simulink model "CRDI_Integrated_Model0707"  (R2019a)
settings: configuration reference "cs1" (kept outside this file)
PreLoadFcn:
  | Configaration_Setting
undefined symbols (not defined in the file or in its folder): AreaOfOrifice_Constant, CcConstant_0, CcConstant_1, Constant_0, Constant_1, Constant_One, Divide_by_100, Error_code_101, Error_code_102, FilterConstant_0, FilterConstant_1, FilterConstant_100, FilterConstant_5, FilterConstant_50, Final_Crank_Angle, Fuel_Discharge, HPPConstant1, HPPConstant2, LPPConstant_0, LPPConstant_1, LPPConstant_10, LPPConstant_3, Main_TgrAng_Inj1, Main_TgrAng_Inj2, Main_TgrAng_Inj3, Main_TgrAng_Inj4, MeterToLiter_Conversion, Orifice_Diameter, Percentage, Pi_value, Post_TgrAng_Inj1, Post_TgrAng_Inj2, Post_TgrAng_Inj3, Post_TgrAng_Inj4, Pre_TgrAng_Inj1, Pre_TgrAng_Inj2, Pre_TgrAng_Inj3, Pre_TgrAng_Inj4, Re_Rounding_Constant, Required_PulseConstant1, Required_PulseConstant2, Required_PulseConstant3, Required_PulseConstant4, resistance_constant, Rounding_Constant_100, Scalling_Factor, Unit_Angle_Compare, Velocity_MulFactor1, Velocity_MulFactor2, Velocity_MulFactor3, Zero_Pulse
libraries: simulink x4
(part 1 of 2)
settings Model: DataDictionary=CRDI_Integrated_Model.sldd  EnableAccessToBaseWorkspace=off  Creator=ADVAIT ELECTRICALS  LastModifiedBy=user
settings ConfigSetRef: SourceName=cs1

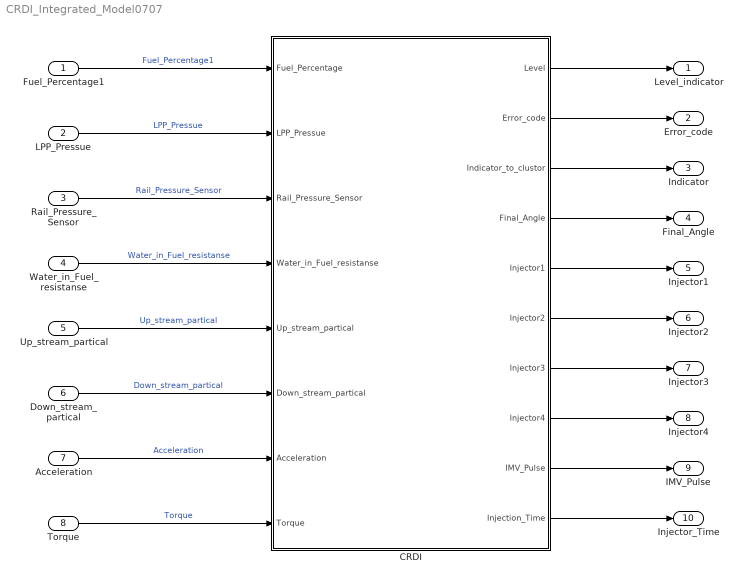
== system CRDI_Integrated_Model0707 ==
  Fuel_Percentage1 : Inport
  LPP_Pressue : Inport  Port=2
  Rail_Pressure_Sensor : Inport  Port=3
  Water_in_Fuel_resistanse : Inport  Port=4
  Up_stream_partical : Inport  Port=5
  Down_stream_partical : Inport  Port=6
  Acceleration : Inport  Port=7
  Torque : Inport  Port=8
  CRDI : Subsystem  TreatAsAtomicUnit=on
  Level_indicator : Outport
  Error_code : Outport  Port=2
  Indicator : Outport  Port=3
  Final_Angle : Outport  Port=4
  Injector1 : Outport  Port=5
  Injector2 : Outport  Port=6
  Injector3 : Outport  Port=7
  Injector4 : Outport  Port=8
  IMV_Pulse : Outport  Port=9
  Injector_Time : Outport  Port=10
  wires:
  LPP_Pressue/1 -> CRDI/2(LPP_Pressue)  "LPP_Pressue"
  Fuel_Percentage1/1 -> CRDI/1(Fuel_Percentage)  "Fuel_Percentage1"
  Rail_Pressure_Sensor/1 -> CRDI/3(Rail_Pressure_Sensor)  "Rail_Pressure_Sensor"
  Up_stream_partical/1 -> CRDI/5(Up_stream_partical)  "Up_stream_partical"
  Water_in_Fuel_resistanse/1 -> CRDI/4(Water_in_Fuel_resistanse)  "Water_in_Fuel_resistanse"
  Down_stream_partical/1 -> CRDI/6(Down_stream_partical)  "Down_stream_partical"
  CRDI/1(Level) -> Level_indicator/1
  CRDI/2(Error_code) -> Error_code/1
  CRDI/3(Indicator_to_clustor) -> Indicator/1
  CRDI/6(Injector2) -> Injector2/1
  CRDI/5(Injector1) -> Injector1/1
  CRDI/4(Final_Angle) -> Final_Angle/1
  CRDI/9(IMV_Pulse) -> IMV_Pulse/1
  CRDI/10(Injection_Time) -> Injector_Time/1
  CRDI/8(Injector4) -> Injector4/1
  CRDI/7(Injector3) -> Injector3/1
  Acceleration/1 -> CRDI/7(Acceleration)  "Acceleration"
  Torque/1 -> CRDI/8(Torque)  "Torque"

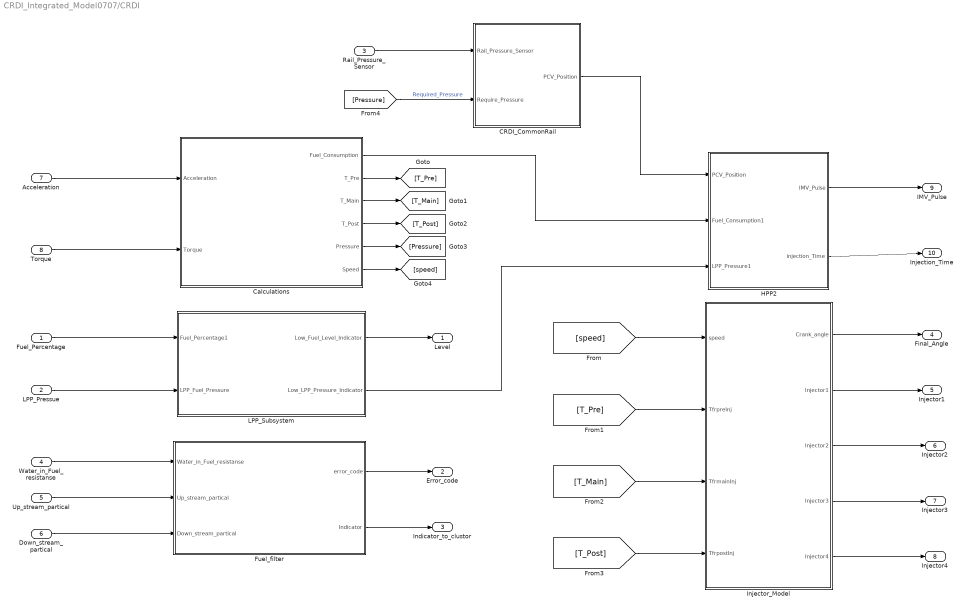
== system CRDI_Integrated_Model0707/CRDI ==
  Fuel_Percentage : Inport
  LPP_Pressue : Inport  Port=2
  Rail_Pressure_Sensor : Inport  Port=3
  Water_in_Fuel_resistanse : Inport  Port=4
  Up_stream_partical : Inport  Port=5
  Down_stream_partical : Inport  Port=6
  Acceleration : Inport  Port=7
  Torque : Inport  Port=8
  CRDI_CommonRail : Subsystem  TreatAsAtomicUnit=on
  Calculations : Subsystem
  Fuel_filter : Subsystem  TreatAsAtomicUnit=on
  HPP2 : Subsystem
  Injector_Model : Subsystem  TreatAsAtomicUnit=on
  LPP_Subsystem : Subsystem  TreatAsAtomicUnit=on
  Level : Outport
  Error_code : Outport  Port=2
  Indicator_to_clustor : Outport  Port=3
  Final_Angle : Outport  Port=4
  Injector1 : Outport  Port=5
  Injector2 : Outport  Port=6
  Injector3 : Outport  Port=7
  Injector4 : Outport  Port=8
  IMV_Pulse : Outport  Port=9
  Injection_Time : Outport  Port=10
  wires:
  CRDI_CommonRail/1(PCV_Position) -> HPP2/1(PCV_Position)
  Fuel_Percentage/1 -> LPP_Subsystem/1(Fuel_Percentage1)
  LPP_Subsystem/1(Low_Fuel_Level_Indicator) -> Level/1
  LPP_Pressue/1 -> LPP_Subsystem/2(LPP_Fuel_Pressure)
  Water_in_Fuel_resistanse/1 -> Fuel_filter/1(Water_in_Fuel_resistanse)
  Down_stream_partical/1 -> Fuel_filter/3(Down_stream_partical)
  Up_stream_partical/1 -> Fuel_filter/2(Up_stream_partical)
  Injector_Model/1(Crank_angle) -> Final_Angle/1
  Injector_Model/5(Injector4) -> Injector4/1
  Injector_Model/2(Injector1) -> Injector1/1
  Injector_Model/3(Injector2) -> Injector2/1
  Injector_Model/4(Injector3) -> Injector3/1
  [speed] -> Injector_Model/1(speed)
  Fuel_filter/1(error_code) -> Error_code/1
  Fuel_filter/2(Indicator) -> Indicator_to_clustor/1
  HPP2/2(injection_Time) -> Injection_Time/1
  HPP2/1(IMV_Pulse) -> IMV_Pulse/1
  LPP_Subsystem/2(Low_LPP_Pressure_Indicator) -> HPP2/3(LPP_Pressure1)
  [T_Pre] -> Injector_Model/2(TfrpreInj)
  [T_Main] -> Injector_Model/3(TfrmainInj)
  [T_Post] -> Injector_Model/4(TfrpostInj)
  Calculations/2(T_Pre) -> [T_Pre]
  Calculations/3(T_Main) -> [T_Main]
  Calculations/4(T_Post) -> [T_Post]
  Calculations/5(Pressure) -> [Pressure]
  Calculations/1(Fuel_Consumption) -> HPP2/2(Fuel_Consumption1)
  Calculations/6(Speed) -> [speed]
  [Pressure] -> CRDI_CommonRail/2(Require_Pressure)  "Required_Pressure"
  Rail_Pressure_Sensor/1 -> CRDI_CommonRail/1(Rail_Pressure_Sensor)
  Acceleration/1 -> Calculations/1(Acceleration)
  Torque/1 -> Calculations/2(Torque)

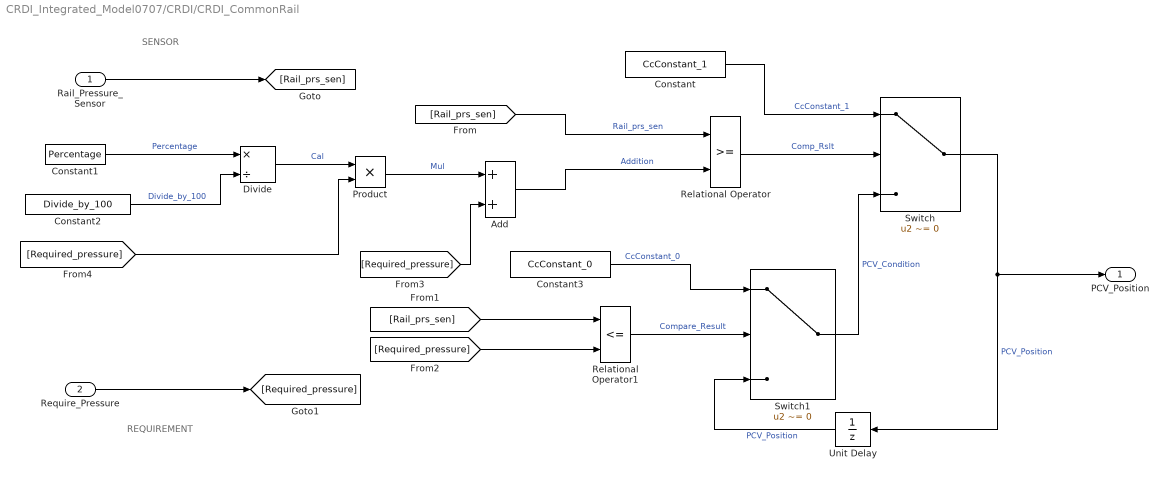
== system CRDI_Integrated_Model0707/CRDI/CRDI_CommonRail ==
  note: REQUIREMENT
  note: SENSOR
  Rail_Pressure_Sensor : Inport
  Require_Pressure : Inport  Port=2
  Add : Sum
  Constant : Constant  Value=CcConstant_1  OutDataTypeStr=boolean
  Constant1 : Constant  Value=Percentage
  Constant2 : Constant  Value=Divide_by_100
  Constant3 : Constant  Value=CcConstant_0  OutDataTypeStr=boolean
  Divide : Product  Inputs=*/  OutDataTypeStr=single
  Product : Product
  Relational Operator : RelationalOperator  OutDataTypeStr=boolean  RndMeth=Simplest
  Relational Operator1 : RelationalOperator  Operator=<=  OutDataTypeStr=boolean  RndMeth=Simplest
  Switch : Switch  Criteria=u2 ~= 0  OutDataTypeStr=boolean
  Switch1 : Switch  Criteria=u2 ~= 0  OutDataTypeStr=boolean
  Unit Delay : UnitDelay  SampleTime=-1  HasFrameUpgradeWarning=on
  PCV_Position : Outport
  wires:
  Constant/1 -> Switch/1  "CcConstant_1"
  Switch/1 -> PCV_Position/1, Unit Delay/1  "PCV_Position"
  Relational Operator/1 -> Switch/2  "Comp_Rslt"
  Unit Delay/1 -> Switch1/3  "PCV_Position"
  Switch1/1 -> Switch/3  "PCV_Condition"
  Product/1 -> Add/1  "Mul"
  Relational Operator1/1 -> Switch1/2  "Compare_Result"
  Add/1 -> Relational Operator/2  "Addition"
  Divide/1 -> Product/1  "Cal"
  Constant3/1 -> Switch1/1  "CcConstant_0"
  Constant1/1 -> Divide/1  "Percentage"
  Constant2/1 -> Divide/2  "Divide_by_100"
  [Rail_prs_sen] -> Relational Operator/1  "Rail_prs_sen"
  Rail_Pressure_Sensor/1 -> [Rail_prs_sen]
  [Rail_prs_sen] -> Relational Operator1/1
  Require_Pressure/1 -> [Required_pressure]
  [Required_pressure] -> Product/2
  [Required_pressure] -> Add/2
  [Required_pressure] -> Relational Operator1/2

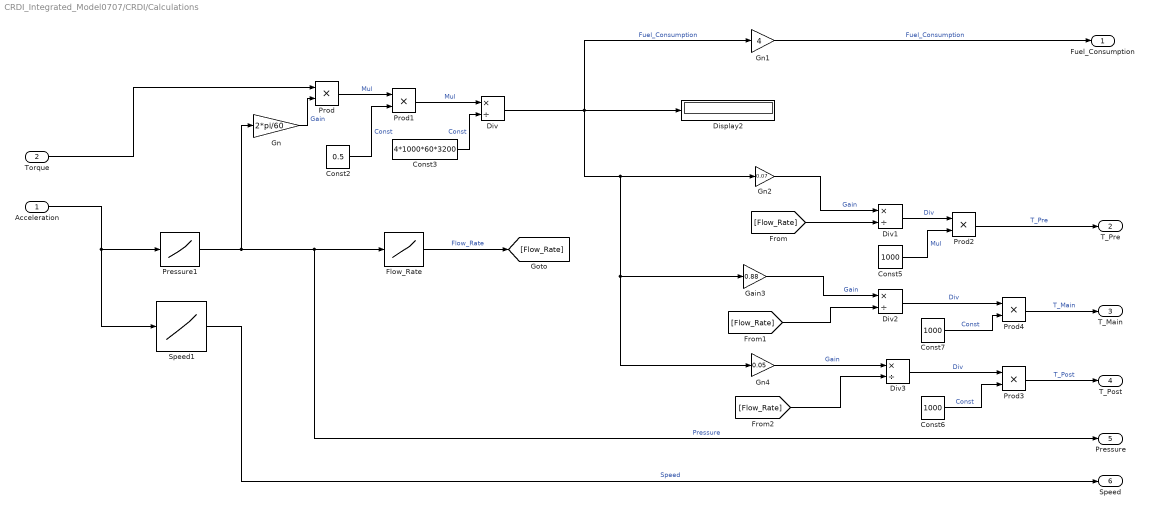
== system CRDI_Integrated_Model0707/CRDI/Calculations ==
  Acceleration : Inport
  Torque : Inport  Port=2
  Const2 : Constant  Value=0.5  OutDataTypeStr=single
  Const3 : Constant  Value=4*1000*60*3200  OutDataTypeStr=single
  Const5 : Constant  Value=1000
  Const6 : Constant  Value=1000  OutDataTypeStr=single
  Const7 : Constant  Value=1000  OutDataTypeStr=single
  Display2 : Display
  Div{,1..3} (4 alike) : Product  Inputs=*/  OutDataTypeStr=single
  Flow_Rate : Lookup_n-D  NumberOfTableDimensions=1  BreakpointsForDimension1=[300 450 600 750 900 1050 1200 1350 1500 1650 1800]  Table=|  InternalRulePriority=Speed  RndMeth=Simplest  InputSameDT=on
      | [0.04780543
      | 0.058549455
      | 0.067607087
      | 0.075587021
      | 0.082801433
      | 0.089435769
      | 0.095610859
      | 0.10141063
      | 0.10689619
      | 0.11211367
      | 0.11709891
      | ]
  Gain3 : Gain  Gain=0.88  OutDataTypeStr=single
  Gn : Gain  Gain=2*pi/60
  Gn1 : Gain  Gain=4  OutDataTypeStr=single
  Gn2 : Gain  Gain=0.07
  Gn4 : Gain  Gain=0.05  OutDataTypeStr=single
  Pressure1 : Lookup_n-D  NumberOfTableDimensions=1  BreakpointsForDimension1=[0 10 20 30 40 50 60 70 80 90 100]  Table=[300 450 600 750 900 1050 1200 1350 1500 1650 1800]  InternalRulePriority=Speed  RndMeth=Simplest  InputSameDT=on
  Prod{,1,3..4} (4 alike) : Product  OutDataTypeStr=single
  Prod2 : Product  OutDataTypeStr=single  SaturateOnIntegerOverflow=on
  Speed1 : Lookup_n-D  NumberOfTableDimensions=1  BreakpointsForDimension1=[0 10 20 30 40 50 60 70 80 90 100]  Table=[800 1040 1280 1520 1760 2000 2240 2480 2720 2960 3200]  InternalRulePriority=Speed  RndMeth=Simplest  InputSameDT=on
  Fuel_Consumption : Outport  OutDataTypeStr=single
  T_Pre : Outport  Port=2  OutDataTypeStr=single
  T_Main : Outport  Port=3  OutDataTypeStr=single
  T_Post : Outport  Port=4  OutDataTypeStr=single
  Pressure : Outport  Port=5  OutDataTypeStr=single
  Speed : Outport  Port=6
  wires:
  Prod/1 -> Prod1/1  "Mul"
  Div2/1 -> Prod4/1  "Div"
  Gn2/1 -> Div1/1  "Gain"
  Const6/1 -> Prod3/2  "Const"
  Pressure1/1 -> Pressure/1, Flow_Rate/1, Gn/1  "Pressure"
  Div/1 -> Gn1/1, Display2/1, Gn4/1, Gain3/1, Gn2/1  "Fuel_Consumption"
  Div3/1 -> Prod3/1  "Div"
  Const2/1 -> Prod1/2  "Const"
  Prod1/1 -> Div/1  "Mul"
  Gn4/1 -> Div3/1  "Gain"
  Const7/1 -> Prod4/2  "Const"
  Acceleration/1 -> Speed1/1, Pressure1/1
  Div1/1 -> Prod2/1  "Div"
  Gn1/1 -> Fuel_Consumption/1  "Fuel_Consumption"
  Prod3/1 -> T_Post/1  "T_Post"
  Prod2/1 -> T_Pre/1  "T_Pre"
  Const3/1 -> Div/2  "Const"
  Gn/1 -> Prod/2  "Gain"
  Const5/1 -> Prod2/2  "Mul"
  Prod4/1 -> T_Main/1  "T_Main"
  Gain3/1 -> Div2/1  "Gain"
  Torque/1 -> Prod/1
  Flow_Rate/1 -> [Flow_Rate]  "Flow_Rate"
  [Flow_Rate] -> Div1/2
  [Flow_Rate] -> Div2/2
  [Flow_Rate] -> Div3/2
  Speed1/1 -> Speed/1  "Speed"

== system CRDI_Integrated_Model0707/CRDI/Fuel_filter ==
  Water_in_Fuel_resistanse : Inport  OutDataTypeStr=single
  Up_stream_partical : Inport  Port=2  OutDataTypeStr=single
  Down_stream_partical : Inport  Port=3  OutDataTypeStr=single
  Calculation : Subsystem
  Condition : Subsystem
  Division_by_0 : Subsystem  TreatAsAtomicUnit=on
  Error_Signal : Subsystem  TreatAsAtomicUnit=on
  Error_code : Subsystem  TreatAsAtomicUnit=on
  On_Delay : Subsystem  TreatAsAtomicUnit=on
  On_delay : Subsystem  TreatAsAtomicUnit=on
  Switch_Condition : Subsystem
  division_by_0 : Subsystem  TreatAsAtomicUnit=on
  error_code : Outport  OutDataTypeStr=single
  Indicator : Outport  Port=2  OutDataTypeStr=boolean
  wires:
  Error_code/1(Error_code) -> error_code/1
  Error_Signal/1(indicator) -> Indicator/1  "Indicator"
  On_Delay/1(error) -> Error_Signal/1(water_error), Error_code/1(water_error)
  On_delay/1(Filter_error) -> Error_code/2(Filter_error), Error_Signal/2(filter_error)
  Down_stream_partical/1 -> Division_by_0/1(Down_stream_partical)
  Water_in_Fuel_resistanse/1 -> Switch_Condition/1(Fuel_Filter)
  Switch_Condition/1(Switch_condition) -> On_Delay/1(switch_condition)
  division_by_0/1(Switch_condition) -> Condition/2(Switch_Condition)
  Condition/1(condition) -> On_delay/1(Switch_condition)
  Up_stream_partical/1 -> Calculation/1(Up_stream_partical)
  Division_by_0/1(Downstream_partical) -> Calculation/2(Down_stream_partical)
  Calculation/1(Add) -> Condition/1(Ad)
  Calculation/2(product) -> division_by_0/1(Beeta_retio)

== system CRDI_Integrated_Model0707/CRDI/HPP2 ==
  PCV_Position : Inport  OutDataTypeStr=boolean
  Fuel_Consumption1 : Inport  Port=2  OutDataTypeStr=single  PortDimensions=1  SampleTime=[0.01,0]
  LPP_Pressure1 : Inport  Port=3  OutDataTypeStr=single  PortDimensions=1  SampleTime=[0.01,0]
  AreaOfOrifice : Subsystem  TreatAsAtomicUnit=on
  Injection_Time_Cal : Subsystem
  Input_Para : Subsystem
  PCV_Position_Action : Subsystem
  Required_Pulse : Subsystem  TreatAsAtomicUnit=on
  Rounding2 : Subsystem  TreatAsAtomicUnit=on
  Rounding3 : Subsystem  Commented=on  TreatAsAtomicUnit=on
  Subsystem1 : Subsystem  Commented=on
  Velocity : Subsystem  TreatAsAtomicUnit=on
  IMV_Pulse : Outport  OutDataTypeStr=boolean  PortDimensions=1  SampleTime=[0.01,0]
  injection_Time : Outport  Port=2  OutDataTypeStr=single  PortDimensions=1  SampleTime=[0.01,0]
  wires:
  Injection_Time_Cal/1(Injection_Time) -> Rounding2/1(In1)
  Fuel_Consumption1/1 -> Injection_Time_Cal/2(Fuel_Consumption)
  Velocity/1(Velocity) -> Input_Para/1(Velocity)
  LPP_Pressure1/1 -> Velocity/1(LPP_Pressurer1)
  Input_Para/1(Multiply11) -> Injection_Time_Cal/1(Flow_Rate)
  AreaOfOrifice/1(Orifice_Area) -> Input_Para/2(Orifice_Area)
  PCV_Position_Action/1(Injector_Time) -> injection_Time/1, Required_Pulse/1(On_Time)
  Rounding2/1(Rounding2) -> PCV_Position_Action/1(Injector_Time1)
  PCV_Position/1 -> PCV_Position_Action/2(PCV_Position)
  Required_Pulse/1(IMV_Pulse) -> IMV_Pulse/1

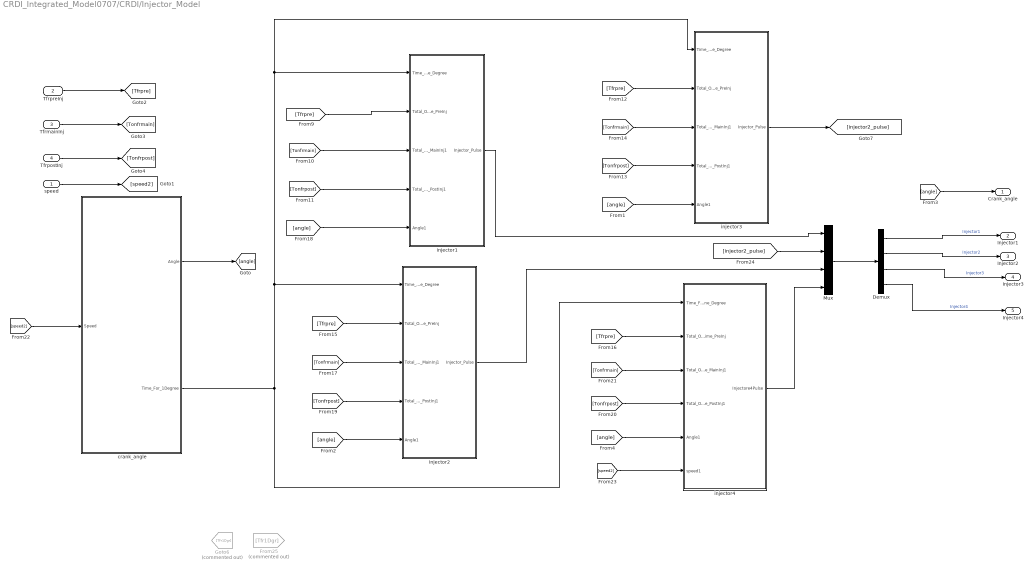
== system CRDI_Integrated_Model0707/CRDI/Injector_Model ==
  speed : Inport  OutDataTypeStr=single
  TfrpreInj : Inport  Port=2  OutDataTypeStr=single
  TfrmainInj : Inport  Port=3  OutDataTypeStr=single
  TfrpostInj : Inport  Port=4  OutDataTypeStr=single
  Demux : Demux
  From25 : From  Commented=on  GotoTag=Tfr1Dgr
  Goto6 : Goto  Commented=on  GotoTag=Tfr1Dgr
  Mux : Mux
  crank_angle : Subsystem  TreatAsAtomicUnit=on
  injector1 : Subsystem  TreatAsAtomicUnit=on
  injector2 : Subsystem  TreatAsAtomicUnit=on
  injector3 : Subsystem  TreatAsAtomicUnit=on
  injector4 : Subsystem  TreatAsAtomicUnit=on
  Crank_angle : Outport
  Injector1 : Outport  Port=2
  Injector2 : Outport  Port=3
  Injector3 : Outport  Port=4
  Injector4 : Outport  Port=5
  wires:
  [Tfrpre] -> injector3/2(Total_On_Time_PreInj)
  [angle] -> injector1/5(Angle1)
  [Tonfrmain] -> injector1/3(Total_On_Time_MainInj1)
  [angle] -> injector4/5(Angle1)
  TfrmainInj/1 -> [Tonfrmain]
  [Tonfrpost] -> injector3/4(Total_On_Time_PostInj1)
  [Tonfrmain] -> injector2/3(Total_On_Time_MainInj1)
  [Tonfrmain] -> injector4/3(Total_On_Time_MainInj1)
  TfrpostInj/1 -> [Tonfrpost]
  [Tfrpre] -> injector2/2(Total_On_Time_PreInj)
  crank_angle/1(Angle) -> [angle]
  crank_angle/2(Time_For_1Degree) -> injector2/1(Time_For_One_Degree), injector3/1(Time_For_One_Degree), injector1/1(Time_For_One_Degree), injector4/1(Time_For_One_Degree)
  [angle] -> injector2/5(Angle1)
  [angle] -> injector3/5(Angle1)
  [Tonfrmain] -> injector3/3(Total_On_Time_MainInj1)
  TfrpreInj/1 -> [Tfrpre]
  [Tonfrpost] -> injector2/4(Total_On_Time_PostInj1)
  [Tfrpre] -> injector4/2(Total_On_Time_PreInj)
  [Tonfrpost] -> injector1/4(Total_On_Time_PostInj1)
  [Tonfrpost] -> injector4/4(Total_On_Time_PostInj1)
  [Tfrpre] -> injector1/2(Total_On_Time_PreInj)
  speed/1 -> [speed2]
  [speed2] -> crank_angle/1(Speed)
  [speed2] -> injector4/6(speed1)
  [angle] -> Crank_angle/1
  injector1/1(Injector_Pulse) -> Mux/1
  injector2/1(Injector_Pulse) -> Mux/3
  injector4/1(Injectore4Pulse) -> Mux/4
  Mux/1 -> Demux/1
  Demux/1 -> Injector1/1  "Injector1"
  Demux/2 -> Injector2/1  "Injector2"
  Demux/3 -> Injector3/1  "Injector3"
  Demux/4 -> Injector4/1  "Injector4"
  injector3/1(Injector_Pulse) -> [injector2_pulse]
  [injector2_pulse] -> Mux/2

== system CRDI_Integrated_Model0707/CRDI/LPP_Subsystem ==
  Fuel_Percentage1 : Inport  OutDataTypeStr=single
  LPP_Fuel_Pressure : Inport  Port=2  OutDataTypeStr=single
  Fuel_Level_Check : Subsystem
  LPP_Pressure_Check : Subsystem
  Low_Fuel_Level_Indicator : Outport
  Low_LPP_Pressure_Indicator : Outport  Port=2
  wires:
  LPP_Fuel_Pressure/1 -> LPP_Pressure_Check/1(pressure)
  Fuel_Percentage1/1 -> Fuel_Level_Check/1(Fuel_percentage)
  Fuel_Level_Check/1(Level_Indicator) -> Low_Fuel_Level_Indicator/1
  LPP_Pressure_Check/1(Pressure_indicator) -> Low_LPP_Pressure_Indicator/1

== system CRDI_Integrated_Model0707/CRDI/Fuel_filter/Calculation ==
  Up_stream_partical : Inport
  Down_stream_partical : Inport  Port=2
  Divide : Product  Inputs=*/  OutDataTypeStr=single  RndMeth=Ceiling
  Subtract : Sum  Inputs=+-  AccumDataTypeStr=single  OutDataTypeStr=single  RndMeth=Ceiling
      settings: AttributesFormatString=|
      | AccumDataTypeStr=%<AccumDataTypeStr>
      | RndMeth=%<RndMeth>
  "sub_1 " : Constant  Value=FilterConstant_1  OutDataTypeStr=single
  Add : Outport
  product : Outport  Port=2
  wires:
  Divide/1 -> product/1, Subtract/1  "product"
  Subtract/1 -> Add/1  "Add"
  "sub_1 "/1 -> Subtract/2  "sub_1"
  Up_stream_partical/1 -> Divide/1
  Down_stream_partical/1 -> Divide/2

== system CRDI_Integrated_Model0707/CRDI/Fuel_filter/Condition ==
  Ad : Inport
  Switch_Condition : Inport  Port=2
  Divide1 : Product  Inputs=*/  OutDataTypeStr=single  RndMeth=Ceiling
  Product : Product  OutDataTypeStr=single  RndMeth=Ceiling
  Relational Operator1 : RelationalOperator  Operator=<=  OutDataTypeStr=boolean  RndMeth=Simplest
  Switch1 : Switch  Criteria=u2 ~= 0  OutDataTypeStr=single
  better_filter : Constant  Value=FilterConstant_0  OutDataTypeStr=single
  filter_efficiency : Constant  Value=FilterConstant_50  OutDataTypeStr=single
  persentage : Constant  Value=FilterConstant_100  OutDataTypeStr=single
  poor_filter : Constant  Value=FilterConstant_1  OutDataTypeStr=single
  condition : Outport
  wires:
  Relational Operator1/1 -> Switch1/2
  filter_efficiency/1 -> Relational Operator1/2  "filter_efficiency"
  Divide1/1 -> Product/1  "Div"
  Switch1/1 -> condition/1  "condition"
  poor_filter/1 -> Switch1/1  "poor_filter"
  Product/1 -> Relational Operator1/1
  better_filter/1 -> Switch1/3  "better_filter"
  persentage/1 -> Product/2  "persentage"
  Ad/1 -> Divide1/1
  Switch_Condition/1 -> Divide1/2

== system CRDI_Integrated_Model0707/CRDI/Fuel_filter/Division_by_0 ==
  Down_stream_partical : Inport  OutDataTypeStr=single
  Relational Operator2 : RelationalOperator  Operator=>  OutDataTypeStr=boolean  RndMeth=Simplest
  Switch2 : Switch  Criteria=u2 ~= 0  OutDataTypeStr=single
  false : Constant  Value=FilterConstant_1  OutDataTypeStr=single
  zero_condition : Constant  Value=FilterConstant_0  OutDataTypeStr=single
  Downstream_partical : Outport  OutDataTypeStr=single
  wires:
  zero_condition/1 -> Relational Operator2/2  "zero_condition"
  Down_stream_partical/1 -> Switch2/1, Relational Operator2/1
  Switch2/1 -> Downstream_partical/1  "Downstream_partical"
  false/1 -> Switch2/3  "false"
  Relational Operator2/1 -> Switch2/2  "Rel_Op"

== system CRDI_Integrated_Model0707/CRDI/Fuel_filter/Error_Signal ==
  water_error : Inport  OutDataTypeStr=boolean
  filter_error : Inport  Port=2  OutDataTypeStr=boolean
  Compare To Constant2 : simulink/Logic and Bit Operations/Compare To Constant  relop===  const=1  OutDataTypeStr=boolean
  OR : Logic  Operator=OR  AllPortsSameDT=off  OutDataTypeStr=boolean
  Switch2 : Switch  Criteria=u2 ~= 0  OutDataTypeStr=boolean
  True_condition : Constant  Value=FilterConstant_1  OutDataTypeStr=single
  false : Constant  Value=FilterConstant_0  OutDataTypeStr=single
  indicator : Outport  OutDataTypeStr=boolean
  wires:
  filter_error/1 -> OR/2
  water_error/1 -> OR/1  "water_error"
  Compare To Constant2/1 -> Switch2/2  "Comp"
  True_condition/1 -> Switch2/1  "True_condition"
  OR/1 -> Compare To Constant2/1  "Or"
  Switch2/1 -> indicator/1  "indicator"
  false/1 -> Switch2/3  "false"

== system CRDI_Integrated_Model0707/CRDI/Fuel_filter/Error_code ==
  water_error : Inport  OutDataTypeStr=boolean
  Filter_error : Inport  Port=2  OutDataTypeStr=boolean
  Compare To Constant1 : simulink/Logic and Bit Operations/Compare To Constant  relop===  const=1  OutDataTypeStr=boolean
  Switch2 : Switch  Criteria=u2 ~= 0  OutDataTypeStr=single
  Switch3 : Switch  Criteria=u2 ~= 0  OutDataTypeStr=single
  false : Constant  Value=FilterConstant_0  OutDataTypeStr=single
  filter_condition_detector : Constant  Value=Error_code_102  OutDataTypeStr=single
  water_detector : Constant  Value=Error_code_101  OutDataTypeStr=int8
  Error_code : Outport  OutDataTypeStr=single
  wires:
  Switch3/1 -> Switch2/3
  filter_condition_detector/1 -> Switch3/1  "Filter_condition"
  Switch2/1 -> Error_code/1  "Error_code"
  water_error/1 -> Compare To Constant1/1  "water_error"
  water_detector/1 -> Switch2/1  "water_detector"
  Filter_error/1 -> Switch3/2  "Filter_error"
  false/1 -> Switch3/3  "false"
  Compare To Constant1/1 -> Switch2/2

== system CRDI_Integrated_Model0707/CRDI/Fuel_filter/On_Delay ==
  switch_condition : Inport  OutDataTypeStr=single
  Add : Sum  AccumDataTypeStr=single  OutDataTypeStr=single
      settings: AttributesFormatString=AccumDataTypeStr=%<AccumDataTypeStr>
  False : Constant  Value=FilterConstant_0  OutDataTypeStr=single
  False1 : Constant  Value=FilterConstant_0  OutDataTypeStr=single
  Relational Operator : RelationalOperator  Operator=>  OutDataTypeStr=boolean  RndMeth=Simplest
  Relational Operator1 : RelationalOperator  Operator=>  OutDataTypeStr=boolean  RndMeth=Simplest
  Switch : Switch  Criteria=u2 ~= 0  OutDataTypeStr=single
  Unit Delay : UnitDelay  SampleTime=-1  HasFrameUpgradeWarning=on
  on_delay_time : Constant  Value=FilterConstant_5  OutDataTypeStr=single
  error : Outport  OutDataTypeStr=boolean
  wires:
  Switch/1 -> Unit Delay/1, Relational Operator/1  "Feedback"
  switch_condition/1 -> Relational Operator1/1, Add/2  "switch_condition"
  False/1 -> Switch/3  "False"
  Add/1 -> Switch/1  "Ad"
  Unit Delay/1 -> Add/1  "Feedback"
  Relational Operator/1 -> error/1  "error"
  on_delay_time/1 -> Relational Operator/2  "on_delay_time"
  Relational Operator1/1 -> Switch/2  "Rel_Op"
  False1/1 -> Relational Operator1/2  "False1"

== system CRDI_Integrated_Model0707/CRDI/Fuel_filter/On_delay ==
  Switch_condition : Inport  OutDataTypeStr=single
  Add : Sum  AccumDataTypeStr=single  OutDataTypeStr=single
      settings: AttributesFormatString=AccumDataTypeStr=%<AccumDataTypeStr>
  False _constant : Constant  Value=FilterConstant_0  OutDataTypeStr=boolean
  False _constant1 : Constant  Value=FilterConstant_0  OutDataTypeStr=boolean
  Relational Operator : RelationalOperator  Operator=>  OutDataTypeStr=boolean  RndMeth=Simplest
  Relational Operator1 : RelationalOperator  Operator=<=  OutDataTypeStr=boolean  RndMeth=Simplest
  Switch : Switch  Criteria=u2 ~= 0  OutDataTypeStr=single
  Unit Delay : UnitDelay  SampleTime=-1  HasFrameUpgradeWarning=on
  on_delay_time : Constant  Value=FilterConstant_5  OutDataTypeStr=single
  Filter_error : Outport  OutDataTypeStr=boolean
  wires:
  on_delay_time/1 -> Relational Operator/2  "on_delay_time"
  Relational Operator/1 -> Filter_error/1  "Filter_error"
  Unit Delay/1 -> Add/1
  Add/1 -> Switch/1
  False _constant/1 -> Switch/3  "False_condition"
  Switch_condition/1 -> Relational Operator1/1, Add/2  "Switch_condition"
  Switch/1 -> Relational Operator/1, Unit Delay/1
  Relational Operator1/1 -> Switch/2
  False _constant1/1 -> Relational Operator1/2  "False_conditions"

== system CRDI_Integrated_Model0707/CRDI/Fuel_filter/Switch_Condition ==
  Fuel_Filter : Inport
  False : Constant  Value=FilterConstant_0  OutDataTypeStr=single
  Relational Operator : RelationalOperator  Operator=<=  OutDataTypeStr=boolean  RndMeth=Simplest
  Switch : Switch  Criteria=u2 ~= 0  OutDataTypeStr=single
  True : Constant  Value=FilterConstant_1  OutDataTypeStr=single
  resistance_constant : Constant  Value=resistance_constant  OutDataTypeStr=single
  Switch_condition : Outport
  wires:
  True/1 -> Switch/1  "True"
  False/1 -> Switch/3  "False"
  Relational Operator/1 -> Switch/2  "Rel_Op"
  resistance_constant/1 -> Relational Operator/2  "resistance_constant"
  Fuel_Filter/1 -> Relational Operator/1
  Switch/1 -> Switch_condition/1  "Switch_condition"

== system CRDI_Integrated_Model0707/CRDI/Fuel_filter/division_by_0 ==
  Beeta_retio : Inport  OutDataTypeStr=single
  Relational Operator2 : RelationalOperator  Operator=>  OutDataTypeStr=boolean  RndMeth=Simplest
  Switch2 : Switch  Criteria=u2 ~= 0  OutDataTypeStr=single
  one_condition : Constant  Value=FilterConstant_1  OutDataTypeStr=single
  zero_condition : Constant  Value=FilterConstant_0  OutDataTypeStr=single
  Switch_condition : Outport  OutDataTypeStr=single
  wires:
  Relational Operator2/1 -> Switch2/2
  one_condition/1 -> Switch2/3  "one_condition"
  Switch2/1 -> Switch_condition/1  "Switch_condition"
  Beeta_retio/1 -> Relational Operator2/1, Switch2/1  "Beeta_retio"
  zero_condition/1 -> Relational Operator2/2  "zero_condition"

== system CRDI_Integrated_Model0707/CRDI/HPP2/AreaOfOrifice ==
  Const : Constant  Value=Pi_value  OutDataTypeStr=single
  Const1 : Constant  Value=AreaOfOrifice_Constant  OutDataTypeStr=single
  Const2 : Constant  Value=Orifice_Diameter  OutDataTypeStr=single
  Div1 : Product  Inputs=*/  OutDataTypeStr=single
  Prod : Product  OutDataTypeStr=single
  Prod1 : Product  OutDataTypeStr=single
  Orifice_Area : Outport  OutDataTypeStr=single
  wires:
  Const2/1 -> Prod/2, Prod/1  "Orifice_Dia"
  Prod1/1 -> Orifice_Area/1  "Orifice_Area"
  Prod/1 -> Prod1/2  "Product"
  Div1/1 -> Prod1/1  "Divide"
  Const1/1 -> Div1/2  "AreaOfOrifice_Constant"
  Const/1 -> Div1/1  "Pi_value"

== system CRDI_Integrated_Model0707/CRDI/HPP2/Injection_Time_Cal ==
  Flow_Rate : Inport
  Fuel_Consumption : Inport  Port=2  OutDataTypeStr=single
  Constant1 : Constant  Value=HPPConstant1  OutDataTypeStr=uint8
  Constant2 : Constant  Value=HPPConstant2  OutDataTypeStr=uint8
  Divide : Product  Inputs=/*  OutDataTypeStr=single
  Flow_Rate_LitperSec : Display
  Product1 : Product  OutDataTypeStr=single
  Relational Operator : RelationalOperator  Operator=>  OutDataTypeStr=boolean  RndMeth=Simplest
  Scalling_Factor : Constant  Value=Scalling_Factor  OutDataTypeStr=single
  Switch : Switch  Criteria=u2 ~= 0  OutDataTypeStr=single
  Injection_Time : Outport
  wires:
  Constant2/1 -> Relational Operator/2  "Constant2"
  Relational Operator/1 -> Switch/2
  Constant1/1 -> Switch/3  "Constant1"
  Switch/1 -> Divide/1
  Fuel_Consumption/1 -> Divide/2
  Flow_Rate/1 -> Flow_Rate_LitperSec/1, Switch/1, Relational Operator/1
  Product1/1 -> Injection_Time/1  "Injection_Time"
  Scalling_Factor/1 -> Product1/2  "Scalling_Factor"
  Divide/1 -> Product1/1

== system CRDI_Integrated_Model0707/CRDI/HPP2/Input_Para ==
  Velocity : Inport
  Orifice_Area : Inport  Port=2
  Constant3 : Constant  Value=MeterToLiter_Conversion
  Display : Display
  Display1 : Display
  Multiply : Gain  Gain=1000000  ParamDataTypeStr=single  OutDataTypeStr=single
  Multiply1 : Gain  Gain=0.000001  ParamDataTypeStr=single  OutDataTypeStr=single
  Product1 : Product  Inputs=3  OutDataTypeStr=single
  Round : Rounding  Operator=round
  Multiply11 : Outport  OutDataTypeStr=single
  wires:
  Round/1 -> Multiply1/1  "Round"
  Constant3/1 -> Product1/3  "MeterToLiter_Conversion"
  Product1/1 -> Display/1, Multiply/1  "Product1"
  Multiply1/1 -> Multiply11/1, Display1/1  "Multiply11"
  Multiply/1 -> Round/1  "Multiply"
  Velocity/1 -> Product1/1
  Orifice_Area/1 -> Product1/2

== system CRDI_Integrated_Model0707/CRDI/HPP2/PCV_Position_Action ==
  Injector_Time1 : Inport
  PCV_Position : Inport  Port=2
  L_O : Logic  Operator=NOT  AllPortsSameDT=off  OutDataTypeStr=boolean
  Switch1 : Switch  Criteria=u2 ~= 0
  Zero_Puls : Constant  Value=Zero_Pulse  OutDataTypeStr=boolean
  Injector_Time : Outport
  wires:
  L_O/1 -> Switch1/2  "PCV_Position"
  Switch1/1 -> Injector_Time/1  "Injector_Time"
  PCV_Position/1 -> L_O/1
  Injector_Time1/1 -> Switch1/1
  Zero_Puls/1 -> Switch1/3  "Zero_Pulse"

== system CRDI_Integrated_Model0707/CRDI/HPP2/Required_Pulse ==
  On_Time : Inport  OutDataTypeStr=single
  Add : Sum  OutDataTypeStr=single
  Constant : Constant  Value=Required_PulseConstant1  OutDataTypeStr=single
  Constant1 : Constant  Value=Required_PulseConstant4  OutDataTypeStr=single
  Constant2 : Constant  Value=Required_PulseConstant2  OutDataTypeStr=boolean
  Constant3 : Constant  Value=Required_PulseConstant3  OutDataTypeStr=boolean
  Multiply : Gain  Gain=100  OutDataTypeStr=single
  Multiply1 : Gain  Gain=0.01  OutDataTypeStr=single
  Relational Operator1 : RelationalOperator  Operator=<=  OutDataTypeStr=boolean  RndMeth=Simplest
  Round : Rounding  Operator=round
  Rounding : Subsystem  Commented=on
  Switch : Switch  Criteria=u2 ~= 0  OutDataTypeStr=boolean
  Switch1 : Switch  Criteria=u2 ~= 0  OutDataTypeStr=single
  TimeFor_Injection1 : Display
  Unit Delay : UnitDelay  SampleTime=-1  HasFrameUpgradeWarning=on
  IMV_Pulse : Outport  OutDataTypeStr=boolean
  wires:
  Round/1 -> Multiply1/1  "Round"
  Multiply/1 -> Round/1  "Multiply"
  [B] -> Switch1/2  "From_RelOp"
  Multiply1/1 -> Relational Operator1/1, Switch1/1  "Multiply1"
  Add/1 -> Multiply/1  "Add"
  On_Time/1 -> Relational Operator1/2
  Constant2/1 -> Switch/1  "Required_PulseConstant2"
  Switch1/1 -> Unit Delay/1  "OP_Switch"
  Constant1/1 -> Switch1/3  "Required_PulseConstant4"
  Unit Delay/1 -> Add/2  "Privious_Value"
  Constant3/1 -> Switch/3  "False_Cond"
  Relational Operator1/1 -> Switch/2, [B]  "Rel_Op"
  Constant/1 -> Add/1  "Constant"
  Switch/1 -> IMV_Pulse/1, TimeFor_Injection1/1  "IMV_Pulse"

== system CRDI_Integrated_Model0707/CRDI/HPP2/Rounding2 ==
  In1 : Inport
  Display : Display
  Display1 : Display
  Multiply : Gain  Gain=100  OutDataTypeStr=single
  Multiply1 : Gain  Gain=0.01  OutDataTypeStr=single
  Round : Rounding  Operator=round
  Rounding2 : Outport  OutDataTypeStr=single
  wires:
  Multiply1/1 -> Display1/1, Rounding2/1  "Rounding2"
  Multiply/1 -> Round/1  "Multiply"
  In1/1 -> Multiply/1, Display/1
  Round/1 -> Multiply1/1  "Round"

== system CRDI_Integrated_Model0707/CRDI/HPP2/Rounding3 ==
  In1 : Inport  OutDataTypeStr=single
  Display : Display
  Display1 : Display
  Multiply : Gain  Gain=1000000  ParamDataTypeStr=single  OutDataTypeStr=single
  Multiply1 : Gain  Gain=0.000001  ParamDataTypeStr=single  OutDataTypeStr=single
  Round : Rounding  Operator=round
  Rounding : Outport  OutDataTypeStr=single
  wires:
  Multiply1/1 -> Rounding/1, Display1/1  "Rounding"
  Multiply/1 -> Round/1
  In1/1 -> Display/1, Multiply/1
  Round/1 -> Multiply1/1

== system CRDI_Integrated_Model0707/CRDI/HPP2/Subsystem1 ==
  In1 : Inport
  In2 : Inport  Port=2
  In3 : Inport  Port=3
  Display : Display
  Display1 : Display
  Multiply : Gain  Gain=1000000  ParamDataTypeStr=single  OutDataTypeStr=single
  Multiply1 : Gain  Gain=0.000001  ParamDataTypeStr=single  OutDataTypeStr=single
  Product1 : Product  Inputs=3  OutDataTypeStr=single
  Round : Rounding  Operator=round
  Rounding : Outport  OutDataTypeStr=single
  wires:
  In2/1 -> Product1/2
  In1/1 -> Product1/1
  Multiply/1 -> Round/1
  Multiply1/1 -> Display1/1, Rounding/1  "Rounding"
  Product1/1 -> Multiply/1, Display/1
  In3/1 -> Product1/3
  Round/1 -> Multiply1/1

== system CRDI_Integrated_Model0707/CRDI/HPP2/Velocity ==
  LPP_Pressurer1 : Inport
  Constant1 : Constant  Value=Velocity_MulFactor3  OutDataTypeStr=double
  Constant3 : Constant  Value=Velocity_MulFactor1  OutDataTypeStr=single
  Constant4 : Constant  Value=Velocity_MulFactor2  OutDataTypeStr=single
  Constant6 : Constant  Value=Fuel_Discharge  OutDataTypeStr=single
  Divide1 : Product  Inputs=*/  OutDataTypeStr=single
  Product : Product
  Product1 : Product  Inputs=3
  Sqr_rt : Sqrt  OutDataTypeStr=single  IntermediateResultsDataTypeStr=single  SaturateOnIntegerOverflow=on
  Velocity : Outport
  wires:
  Sqr_rt/1 -> Product/2  "Sqr_rt"
  Product/1 -> Velocity/1  "Velocity"
  Constant4/1 -> Product1/3  "Velocity_MulFactor2"
  Product1/1 -> Divide1/1  "Product1"
  Constant1/1 -> Product/1  "Velocity_MulFactor3"
  Constant6/1 -> Divide1/2  "Fuel_Discharge"
  Constant3/1 -> Product1/2  "Velocity_MulFactor1"
  LPP_Pressurer1/1 -> Product1/1
  Divide1/1 -> Sqr_rt/1  "Divide1"

== system CRDI_Integrated_Model0707/CRDI/Injector_Model/crank_angle ==
  Speed : Inport  OutDataTypeStr=single
  Subsystem : Subsystem
  Subsystem1 : Subsystem
  Angle : Outport  OutDataTypeStr=single
  Time_For_1Degree : Outport  Port=2  OutDataTypeStr=single
  wires:
  Subsystem/1(Final_Angle) -> Angle/1
  Speed/1 -> Subsystem1/1(Speed)
  Subsystem1/1(Time_For_1_Degree) -> Time_For_1Degree/1
  Subsystem1/2(Angle_Increment) -> Subsystem/Enable

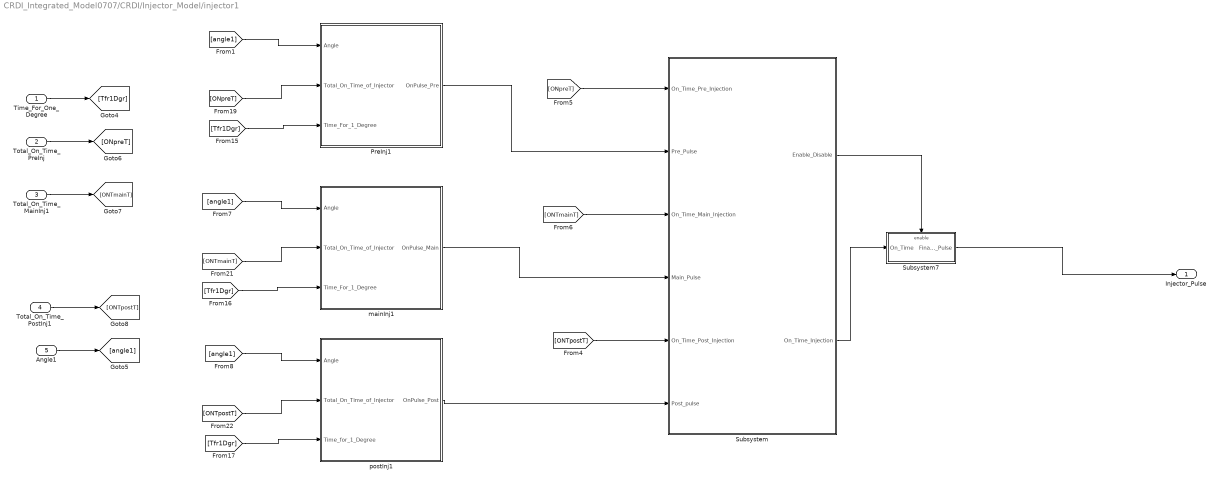
== system CRDI_Integrated_Model0707/CRDI/Injector_Model/injector1 ==
  Time_For_One_Degree : Inport  OutDataTypeStr=single
  Total_On_Time_PreInj : Inport  Port=2  OutDataTypeStr=single
  Total_On_Time_MainInj1 : Inport  Port=3  OutDataTypeStr=single
  Total_On_Time_PostInj1 : Inport  Port=4  OutDataTypeStr=single
  Angle1 : Inport  Port=5  OutDataTypeStr=single
  PreInj1 : Subsystem
  Subsystem : Subsystem
  Subsystem7 : Subsystem
  mainInj1 : Subsystem
  postInj1 : Subsystem
  Injector_Pulse : Outport
  wires:
  postInj1/1(OnPulse_Post) -> Subsystem/6(Post_pulse)
  mainInj1/1(OnPulse_Main) -> Subsystem/4(Main_Pulse)
  PreInj1/1(OnPulse_Pre) -> Subsystem/2(Pre_Pulse)
  [ONTmainT] -> Subsystem/3(On_Time_Main_Injection)
  [ONpreT] -> Subsystem/1(On_Time_Pre_Injection)
  [ONTpostT] -> Subsystem/5(On_Time_Post_Injection)
  Subsystem/2(On_Time_Injection) -> Subsystem7/1(On_Time)
  Subsystem/1(Enable_Disable) -> Subsystem7/Enable
  [angle1] -> PreInj1/1(Angle)
  [angle1] -> postInj1/1(Angle)
  Total_On_Time_PostInj1/1 -> [ONTpostT]
  [ONpreT] -> PreInj1/2(Total_On_Time_of_Injector)
  Total_On_Time_PreInj/1 -> [ONpreT]
  Time_For_One_Degree/1 -> [Tfr1Dgr]
  [Tfr1Dgr] -> PreInj1/3(Time_For_1_Degree)
  [ONTmainT] -> mainInj1/2(Total_On_Time_of_Injector)
  Angle1/1 -> [angle1]
  [ONTpostT] -> postInj1/2(Total_On_Time_of_Injector)
  [Tfr1Dgr] -> mainInj1/3(Time_For_1_Degree)
  Total_On_Time_MainInj1/1 -> [ONTmainT]
  [angle1] -> mainInj1/1(Angle)
  Subsystem7/1(Final_Inj_Pulse) -> Injector_Pulse/1
  [Tfr1Dgr] -> postInj1/3(Time_for_1_Degree)

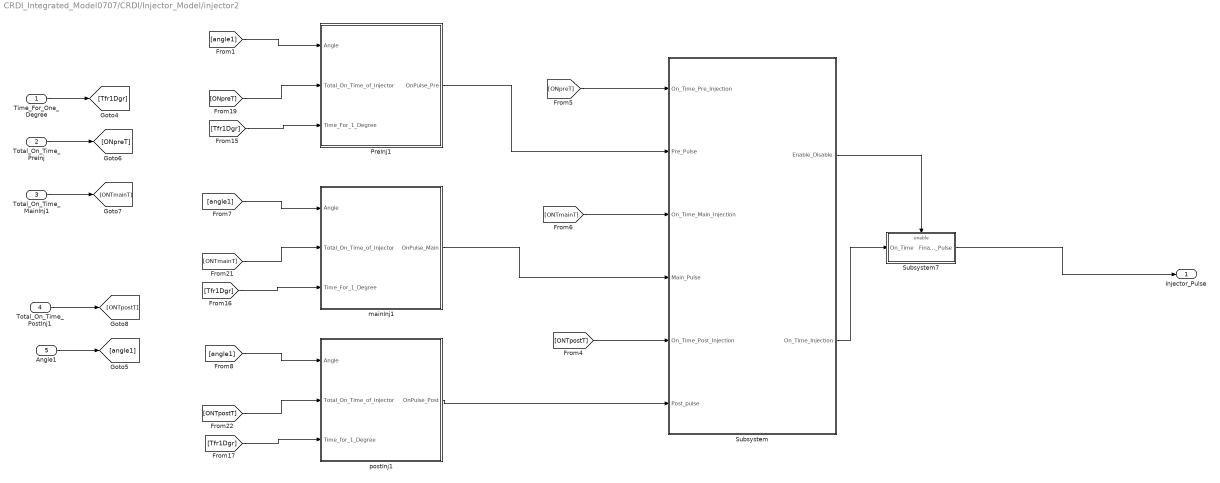
== system CRDI_Integrated_Model0707/CRDI/Injector_Model/injector2 ==
  Time_For_One_Degree : Inport  OutDataTypeStr=single
  Total_On_Time_PreInj : Inport  Port=2  OutDataTypeStr=single
  Total_On_Time_MainInj1 : Inport  Port=3  OutDataTypeStr=single
  Total_On_Time_PostInj1 : Inport  Port=4  OutDataTypeStr=single
  Angle1 : Inport  Port=5  OutDataTypeStr=single
  PreInj1 : Subsystem
  Subsystem : Subsystem
  Subsystem7 : Subsystem
  mainInj1 : Subsystem
  postInj1 : Subsystem
  Injector_Pulse : Outport
  wires:
  postInj1/1(OnPulse_Post) -> Subsystem/6(Post_pulse)
  mainInj1/1(OnPulse_Main) -> Subsystem/4(Main_Pulse)
  PreInj1/1(OnPulse_Pre) -> Subsystem/2(Pre_Pulse)
  [ONTmainT] -> Subsystem/3(On_Time_Main_Injection)
  [ONpreT] -> Subsystem/1(On_Time_Pre_Injection)
  [ONTpostT] -> Subsystem/5(On_Time_Post_Injection)
  Subsystem/2(On_Time_Injection) -> Subsystem7/1(On_Time)
  Subsystem/1(Enable_Disable) -> Subsystem7/Enable
  [angle1] -> PreInj1/1(Angle)
  [angle1] -> postInj1/1(Angle)
  Total_On_Time_PostInj1/1 -> [ONTpostT]
  [ONpreT] -> PreInj1/2(Total_On_Time_of_Injector)
  Total_On_Time_PreInj/1 -> [ONpreT]
  Time_For_One_Degree/1 -> [Tfr1Dgr]
  [Tfr1Dgr] -> PreInj1/3(Time_For_1_Degree)
  [ONTmainT] -> mainInj1/2(Total_On_Time_of_Injector)
  Angle1/1 -> [angle1]
  [ONTpostT] -> postInj1/2(Total_On_Time_of_Injector)
  [Tfr1Dgr] -> mainInj1/3(Time_For_1_Degree)
  Total_On_Time_MainInj1/1 -> [ONTmainT]
  [angle1] -> mainInj1/1(Angle)
  Subsystem7/1(Final_Inj_Pulse) -> Injector_Pulse/1
  [Tfr1Dgr] -> postInj1/3(Time_for_1_Degree)

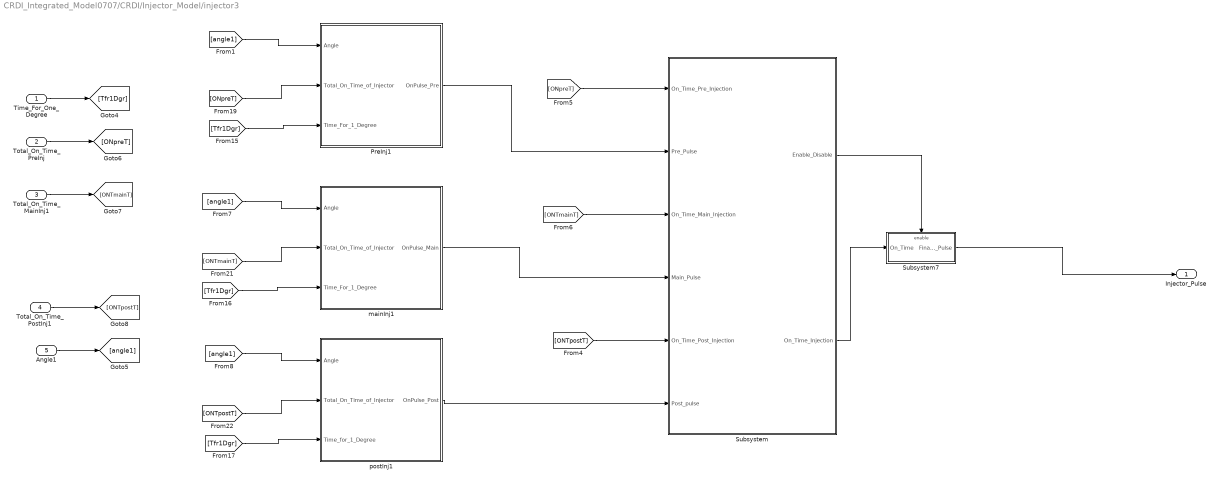
== system CRDI_Integrated_Model0707/CRDI/Injector_Model/injector3 ==
  Time_For_One_Degree : Inport  OutDataTypeStr=single
  Total_On_Time_PreInj : Inport  Port=2  OutDataTypeStr=single
  Total_On_Time_MainInj1 : Inport  Port=3  OutDataTypeStr=single
  Total_On_Time_PostInj1 : Inport  Port=4  OutDataTypeStr=single
  Angle1 : Inport  Port=5  OutDataTypeStr=single
  PreInj1 : Subsystem
  Subsystem : Subsystem
  Subsystem7 : Subsystem
  mainInj1 : Subsystem
  postInj1 : Subsystem
  Injector_Pulse : Outport
  wires:
  postInj1/1(OnPulse_Post) -> Subsystem/6(Post_pulse)
  mainInj1/1(OnPulse_Main) -> Subsystem/4(Main_Pulse)
  PreInj1/1(OnPulse_Pre) -> Subsystem/2(Pre_Pulse)
  [ONTmainT] -> Subsystem/3(On_Time_Main_Injection)
  [ONpreT] -> Subsystem/1(On_Time_Pre_Injection)
  [ONTpostT] -> Subsystem/5(On_Time_Post_Injection)
  Subsystem/2(On_Time_Injection) -> Subsystem7/1(On_Time)
  Subsystem/1(Enable_Disable) -> Subsystem7/Enable
  [angle1] -> PreInj1/1(Angle)
  [angle1] -> postInj1/1(Angle)
  Total_On_Time_PostInj1/1 -> [ONTpostT]
  [ONpreT] -> PreInj1/2(Total_On_Time_of_Injector)
  Total_On_Time_PreInj/1 -> [ONpreT]
  Time_For_One_Degree/1 -> [Tfr1Dgr]
  [Tfr1Dgr] -> PreInj1/3(Time_For_1_Degree)
  [ONTmainT] -> mainInj1/2(Total_On_Time_of_Injector)
  Angle1/1 -> [angle1]
  [ONTpostT] -> postInj1/2(Total_On_Time_of_Injector)
  [Tfr1Dgr] -> mainInj1/3(Time_For_1_Degree)
  Total_On_Time_MainInj1/1 -> [ONTmainT]
  [angle1] -> mainInj1/1(Angle)
  Subsystem7/1(Final_Inj_Pulse) -> Injector_Pulse/1
  [Tfr1Dgr] -> postInj1/3(Time_for_1_Degree)

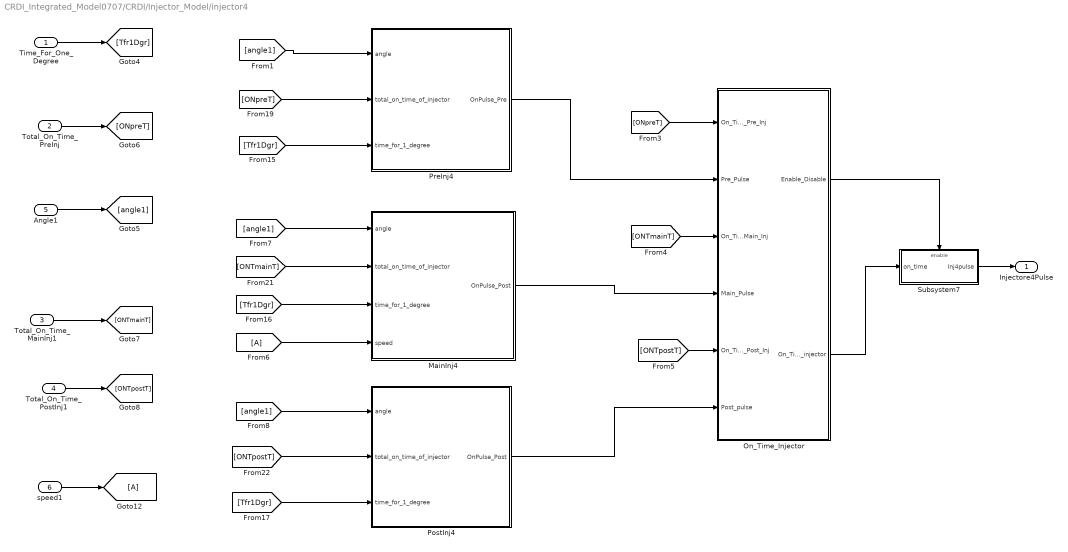
== system CRDI_Integrated_Model0707/CRDI/Injector_Model/injector4 ==
  Time_For_One_Degree : Inport  OutDataTypeStr=single
  Total_On_Time_PreInj : Inport  Port=2  OutDataTypeStr=single
  Total_On_Time_MainInj1 : Inport  Port=3  OutDataTypeStr=single
  Total_On_Time_PostInj1 : Inport  Port=4  OutDataTypeStr=single
  Angle1 : Inport  Port=5  OutDataTypeStr=single
  speed1 : Inport  Port=6  OutDataTypeStr=single
  MainInj4 : Subsystem
  On_Time_Injector : Subsystem
  PostInj4 : Subsystem
  PreInj4 : Subsystem
  Subsystem7 : Subsystem
  Injectore4Pulse : Outport
  wires:
  [angle1] -> PostInj4/1(angle)
  Total_On_Time_PostInj1/1 -> [ONTpostT]
  [ONpreT] -> PreInj4/2(total_on_time_of_injector)
  Total_On_Time_PreInj/1 -> [ONpreT]
  Time_For_One_Degree/1 -> [Tfr1Dgr]
  [Tfr1Dgr] -> PreInj4/3(time_for_1_degree)
  [ONTmainT] -> MainInj4/2(total_on_time_of_injector)
  Angle1/1 -> [angle1]
  [ONTpostT] -> PostInj4/2(total_on_time_of_injector)
  [Tfr1Dgr] -> MainInj4/3(time_for_1_degree)
  Total_On_Time_MainInj1/1 -> [ONTmainT]
  [angle1] -> MainInj4/1(angle)
  [A] -> MainInj4/4(speed)
  speed1/1 -> [A]
  [ONpreT] -> On_Time_Injector/1(On_Time_Pre_Inj)
  [ONTmainT] -> On_Time_Injector/3(On_Time_Main_Inj)
  [ONTpostT] -> On_Time_Injector/5(On_Time_Post_Inj)
  PreInj4/1(OnPulse_Pre) -> On_Time_Injector/2(Pre_Pulse)
  MainInj4/1(OnPulse_Post) -> On_Time_Injector/4(Main_Pulse)
  PostInj4/1(OnPulse_Post) -> On_Time_Injector/6(Post_pulse)
  Subsystem7/1(Inj4pulse) -> Injectore4Pulse/1
  On_Time_Injector/1(Enable_Disable) -> Subsystem7/Enable
  On_Time_Injector/2(On_Time_injector) -> Subsystem7/1(on_time)
  [Tfr1Dgr] -> PostInj4/3(time_for_1_degree)
  [angle1] -> PreInj4/1(angle)

== system CRDI_Integrated_Model0707/CRDI/LPP_Subsystem/Fuel_Level_Check ==
  Fuel_percentage : Inport  OutDataTypeStr=single
  Compare To Constant : simulink/Logic and Bit Operations/Compare To Constant  relop=>=  const=LPPConstant_10  OutDataTypeStr=boolean
  Constant : Constant  Value=LPPConstant_0  OutDataTypeStr=boolean
  Constant1 : Constant  Value=LPPConstant_1  OutDataTypeStr=boolean
  Switch : Switch  Criteria=u2 ~= 0  OutDataTypeStr=boolean
  Level_Indicator : Outport  OutDataTypeStr=boolean
  wires:
  Switch/1 -> Level_Indicator/1  "Level_Indicator"
  Constant1/1 -> Switch/3  "Constant_1"
  Constant/1 -> Switch/1  "Contant_0"
  Compare To Constant/1 -> Switch/2  "compare"
  Fuel_percentage/1 -> Compare To Constant/1

== system CRDI_Integrated_Model0707/CRDI/LPP_Subsystem/LPP_Pressure_Check ==
  pressure : Inport  OutDataTypeStr=single
  Compare To Constant : simulink/Logic and Bit Operations/Compare To Constant  relop=>=  const=LPPConstant_3  OutDataTypeStr=boolean
  Constant : Constant  Value=LPPConstant_0  OutDataTypeStr=single
  Constant1 : Constant  Value=LPPConstant_1  OutDataTypeStr=single
  Switch : Switch  Criteria=u2 ~= 0  OutDataTypeStr=single
  Pressure_indicator : Outport  OutDataTypeStr=single
  wires:
  pressure/1 -> Compare To Constant/1
  Compare To Constant/1 -> Switch/2  "compare"
  Constant/1 -> Switch/1  "Constant_0"
  Constant1/1 -> Switch/3  "Constant_1"
  Switch/1 -> Pressure_indicator/1  "Pressure_indicator"

== system CRDI_Integrated_Model0707/CRDI/HPP2/Required_Pulse/Rounding ==
  Add1 : Inport
  Multiply2 : Gain  Gain=100  OutDataTypeStr=single
  Multiply3 : Gain  Gain=0.01  OutDataTypeStr=single
  Round1 : Rounding  Operator=round
  Out1 : Outport
  wires:
  Multiply3/1 -> Out1/1  "Multiply1"
  Multiply2/1 -> Round1/1  "Multiply"
  Add1/1 -> Multiply2/1
  Round1/1 -> Multiply3/1  "Round"

== system CRDI_Integrated_Model0707/CRDI/Injector_Model/crank_angle/Subsystem ==
  Enable : EnablePort
  Add1 : Sum  AccumDataTypeStr=single
      settings: AttributesFormatString=AccumDataTypeStr=%<AccumDataTypeStr>
  Constant1 : Constant  Value=Constant_0  OutDataTypeStr=single
  Constant2 : Constant  Value=Final_Crank_Angle  OutDataTypeStr=single
  Constant6 : Constant  Value=Constant_1  OutDataTypeStr=single
  Relational Operator : RelationalOperator  Operator=<  OutDataTypeStr=boolean  RndMeth=Simplest
  Switch1 : Switch  Criteria=u2 ~= 0
  Unit Delay1 : UnitDelay  SampleTime=-1  HasFrameUpgradeWarning=on
  Final_Angle : Outport  OutDataTypeStr=single
  wires:
  Unit Delay1/1 -> Relational Operator/1, Add1/1
  Switch1/1 -> Final_Angle/1, Unit Delay1/1  "Final_Angle"
  Constant6/1 -> Add1/2  "one"
  Add1/1 -> Switch1/1
  Constant1/1 -> Switch1/3  "zero"
  Constant2/1 -> Relational Operator/2  "Final_Crank_Angle"
  Relational Operator/1 -> Switch1/2

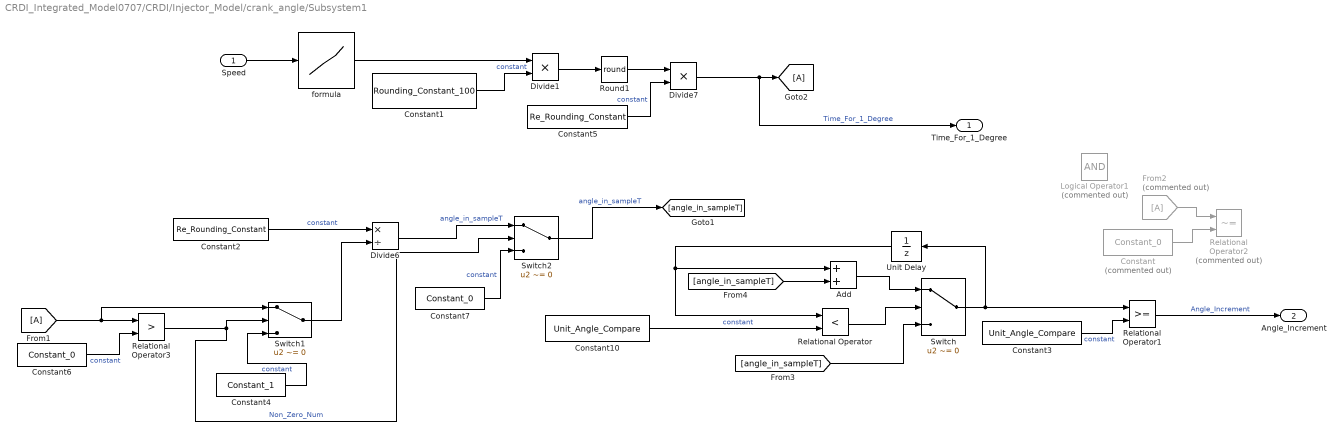
== system CRDI_Integrated_Model0707/CRDI/Injector_Model/crank_angle/Subsystem1 ==
  Speed : Inport  OutDataTypeStr=single
  Add : Sum  AccumDataTypeStr=single
      settings: AttributesFormatString=AccumDataTypeStr=%<AccumDataTypeStr>
  Constant : Constant  Commented=on  Value=Constant_0  OutDataTypeStr=single
  Constant1 : Constant  Value=Rounding_Constant_100  OutDataTypeStr=single
  Constant10 : Constant  Value=Unit_Angle_Compare  OutDataTypeStr=single
  Constant2 : Constant  Value=Re_Rounding_Constant  OutDataTypeStr=single
  Constant3 : Constant  Value=Unit_Angle_Compare  OutDataTypeStr=single
  Constant4 : Constant  Value=Constant_1
  Constant5 : Constant  Value=Re_Rounding_Constant  OutDataTypeStr=single
  Constant6 : Constant  Value=Constant_0
  Constant7 : Constant  Value=Constant_0
  Divide1 : Product  Inputs=**  OutDataTypeStr=single  RndMeth=Convergent  SaturateOnIntegerOverflow=on  LockScale=on
  Divide6 : Product  Inputs=*/  OutDataTypeStr=single
  Divide7 : Product  Inputs=**  OutDataTypeStr=single  RndMeth=Convergent  SaturateOnIntegerOverflow=on  LockScale=on
  From2 : From  Commented=on
  Logical Operator1 : Logic  Commented=on  AllPortsSameDT=off  OutDataTypeStr=boolean
  Relational Operator : RelationalOperator  Operator=<  OutDataTypeStr=boolean  RndMeth=Simplest
  Relational Operator1 : RelationalOperator  OutDataTypeStr=boolean  RndMeth=Simplest
  Relational Operator2 : RelationalOperator  Commented=on  Operator=~=  OutDataTypeStr=boolean  RndMeth=Simplest
  Relational Operator3 : RelationalOperator  Operator=>  OutDataTypeStr=boolean  RndMeth=Simplest
  Round1 : Rounding  Operator=round
      settings: AttributesFormatString=Operator=%<Operator>
  Switch : Switch  Criteria=u2 ~= 0
  Switch1 : Switch  Criteria=u2 ~= 0
  Switch2 : Switch  Criteria=u2 ~= 0
  Unit Delay : UnitDelay  SampleTime=-1  HasFrameUpgradeWarning=on
  formula : Lookup_n-D  NumberOfTableDimensions=1  BreakpointsForDimension1=[0 800 1040 1280 1520 1760 2000 2240 2480 2720 2960 3200]  Table=[0 0.1 0.08 0.07 0.05 0.05 0.04 0.04 0.03 0.03 0.03 0.03]  InternalRulePriority=Speed  RndMeth=Simplest  InputSameDT=on
      settings: AttributesFormatString=RndMeth=%<RndMeth>
  Time_For_1_Degree : Outport  OutDataTypeStr=single
  Angle_Increment : Outport  Port=2
  wires:
  formula/1 -> Divide1/1
  Unit Delay/1 -> Add/1, Relational Operator/1
  Switch/1 -> Relational Operator1/1, Unit Delay/1
  From2/1 -> Relational Operator2/1
  [angle_in_sampleT] -> Switch/3
  Constant2/1 -> Divide6/1  "constant"
  Constant3/1 -> Relational Operator1/2  "constant"
  Constant5/1 -> Divide7/2  "constant"
  Divide7/1 -> Time_For_1_Degree/1, [A]  "Time_For_1_Degree"
  Add/1 -> Switch/1
  Constant10/1 -> Relational Operator/2  "constant"
  Relational Operator/1 -> Switch/2
  Switch1/1 -> Divide6/2
  [angle_in_sampleT] -> Add/2
  Constant/1 -> Relational Operator2/2
  Speed/1 -> formula/1
  Constant4/1 -> Switch1/3  "constant"
  Round1/1 -> Divide7/1
  Divide1/1 -> Round1/1
  Constant1/1 -> Divide1/2  "constant"
  Relational Operator1/1 -> Angle_Increment/1  "Angle_Increment"
  Constant6/1 -> Relational Operator3/2  "constant"
  [A] -> Switch1/1, Relational Operator3/1
  Relational Operator3/1 -> Switch1/2, Switch2/2  "Non_Zero_Num"
  Switch2/1 -> [angle_in_sampleT]  "angle_in_sampleT"
  Divide6/1 -> Switch2/1  "angle_in_sampleT"
  Constant7/1 -> Switch2/3  "constant"

== system CRDI_Integrated_Model0707/CRDI/Injector_Model/injector1/PreInj1 ==
  Angle : Inport  OutDataTypeStr=single
  Total_On_Time_of_Injector : Inport  Port=2  OutDataTypeStr=single
  Time_For_1_Degree : Inport  Port=3  OutDataTypeStr=single
  Add : Sum  AccumDataTypeStr=single
      settings: AttributesFormatString=AccumDataTypeStr=%<AccumDataTypeStr>
  Constant : Constant  Value=Constant_0
  Constant1 : Constant  Value=Constant_1
  Constant2 : Constant  Value=Pre_TgrAng_Inj1  OutDataTypeStr=single
  Constant6 : Constant  Value=Constant_0
  Divide : Product  Inputs=*/  OutDataTypeStr=single
  Logical Operator : Logic  Inputs=3  AllPortsSameDT=off  OutDataTypeStr=boolean
  Relational Operator : RelationalOperator  OutDataTypeStr=boolean  RndMeth=Simplest
  Relational Operator1 : RelationalOperator  Operator=<=  OutDataTypeStr=boolean  RndMeth=Simplest
  Relational Operator2 : RelationalOperator  Operator=>  OutDataTypeStr=boolean  RndMeth=Simplest
  Relational Operator3 : RelationalOperator  Operator=>  OutDataTypeStr=boolean  RndMeth=Simplest
  Switch : Switch  Criteria=u2 ~= 0
  OnPulse_Pre : Outport
  wires:
  Time_For_1_Degree/1 -> Relational Operator3/1, Switch/1
  Constant1/1 -> Switch/3  "constant"
  Switch/1 -> Divide/2  "Time_Of_1_Degree"
  Constant2/1 -> [TrigerAngle], Add/1  "TrigerAngle"
  [TrigerAngle] -> Relational Operator/2
  [onTinj] -> Relational Operator2/1
  Total_On_Time_of_Injector/1 -> [onTinj], Divide/1
  Constant/1 -> Relational Operator2/2  "constant"
  Relational Operator2/1 -> Logical Operator/3  "Speed_Zero_Or_Not"
  Logical Operator/1 -> OnPulse_Pre/1  "OnPulse_Pre"
  Relational Operator1/1 -> Logical Operator/2  "Firing_Angle_Off"
  Relational Operator/1 -> Logical Operator/1  "Firing_Angle_start"
  Add/1 -> Relational Operator1/2  "Total_On_Degree"
  Angle/1 -> Relational Operator1/1, Relational Operator/1
  Divide/1 -> Add/2  "Time_For_On_Pulse"
  Relational Operator3/1 -> Switch/2  "Non_Zero_Num"
  Constant6/1 -> Relational Operator3/2  "constant"

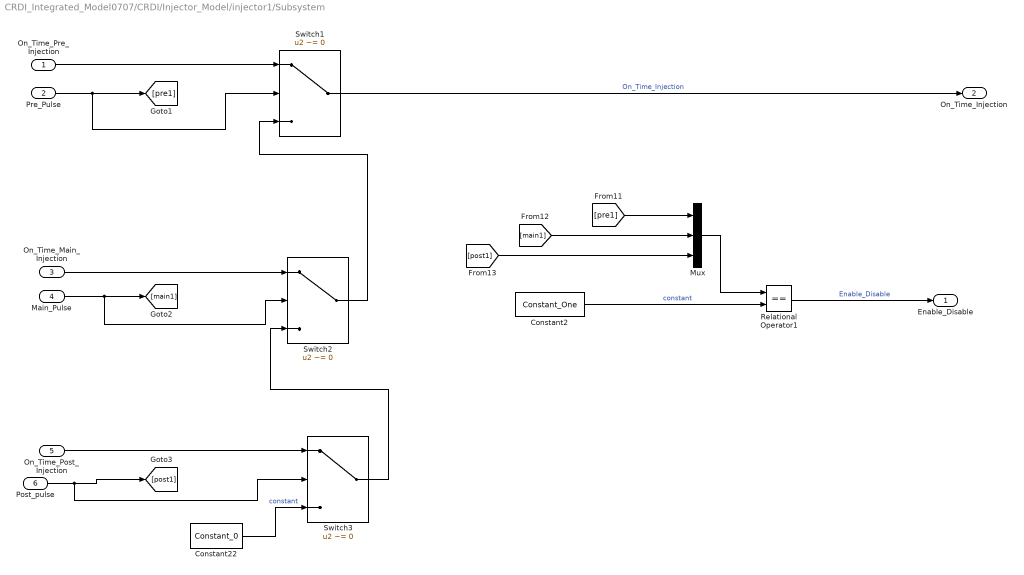
== system CRDI_Integrated_Model0707/CRDI/Injector_Model/injector1/Subsystem ==
  On_Time_Pre_Injection : Inport
  Pre_Pulse : Inport  Port=2
  On_Time_Main_Injection : Inport  Port=3
  Main_Pulse : Inport  Port=4
  On_Time_Post_Injection : Inport  Port=5
  Post_pulse : Inport  Port=6
  Constant2 : Constant  Value=Constant_One  OutDataTypeStr=single
  Constant22 : Constant  Value=Constant_0  OutDataTypeStr=single
  Mux : Mux  Inputs=3
  Relational Operator1 : RelationalOperator  Operator===  OutDataTypeStr=boolean  RndMeth=Simplest
  Switch1 : Switch  Criteria=u2 ~= 0
  Switch2 : Switch  Criteria=u2 ~= 0
  Switch3 : Switch  Criteria=u2 ~= 0
  Enable_Disable : Outport
  On_Time_Injection : Outport  Port=2
  wires:
  Post_pulse/1 -> [post1], Switch3/2
  On_Time_Post_Injection/1 -> Switch3/1
  Main_Pulse/1 -> [main1], Switch2/2
  On_Time_Main_Injection/1 -> Switch2/1
  Pre_Pulse/1 -> [pre1], Switch1/2
  On_Time_Pre_Injection/1 -> Switch1/1
  Switch1/1 -> On_Time_Injection/1  "On_Time_Injection"
  Relational Operator1/1 -> Enable_Disable/1  "Enable_Disable"
  Constant22/1 -> Switch3/3  "constant"
  [main1] -> Mux/2
  Constant2/1 -> Relational Operator1/2  "constant"
  Switch3/1 -> Switch2/3
  Switch2/1 -> Switch1/3
  Mux/1 -> Relational Operator1/1
  [pre1] -> Mux/1
  [post1] -> Mux/3

== system CRDI_Integrated_Model0707/CRDI/Injector_Model/injector1/Subsystem7 ==
  On_Time : Inport
  Enable : EnablePort  StatesWhenEnabling=reset  PropagateVarSize=During execution
  Add : Sum  AccumDataTypeStr=single
      settings: AttributesFormatString=AccumDataTypeStr=%<AccumDataTypeStr>
  Constant : Constant  Value=Re_Rounding_Constant  OutDataTypeStr=single
  Relational Operator : RelationalOperator  Operator=<=  OutDataTypeStr=boolean  RndMeth=Simplest
  Subsystem : Subsystem  Commented=on
  Unit Delay : UnitDelay  SampleTime=-1  HasFrameUpgradeWarning=on
  Final_Inj_Pulse : Outport  OutDataTypeStr=boolean
  wires:
  Relational Operator/1 -> Final_Inj_Pulse/1  "Final_Inj_Pulse"
  Unit Delay/1 -> Add/1
  Constant/1 -> Add/2  "constant"
  Add/1 -> Relational Operator/1, Unit Delay/1
  On_Time/1 -> Relational Operator/2
